simulink model "pidController"  (R2024a)
settings: Solver=VariableStepAuto  StartTime=0.0  StopTime=0.1  MaxStep=0.001  RelTol=1e-3
values from neighbouring files (symbols this model uses):
  C2 = 1e-7    (= 1e-07)    [plotPidController.m]
  C3 = 1e-6    (= 1e-06)    [plotPidController.m]
  R6 = 2e3    (= 2000)    [plotPidController.m]
settings Model: Creator=janho  LastModifiedBy=janho

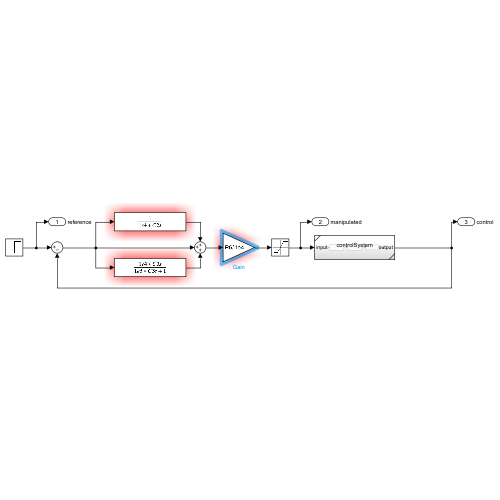
[thumbnail: Simulink's stored preview of the top-level diagram]
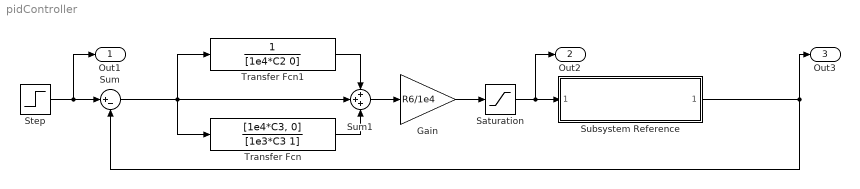
== system pidController ==
  Gain : Gain  Gain=R6/1e4
  Saturation : Saturate  UpperLimit=12  LowerLimit=-12
  Step : Step  Time=0  After=5  SampleTime=0
  Subsystem Reference : Subsystem  ReferencedSubsystem=controlSystem
  Sum : Sum  Inputs=|+-
  Sum1 : Sum  Inputs=+++
  Transfer Fcn : TransferFcn  Numerator=[1e4*C3, 0]  Denominator=[1e3*C3 1]
  Transfer Fcn1 : TransferFcn  Denominator=[1e4*C2 0]
  Out1 : Outport  SignalName=reference
  Out2 : Outport  Port=2  SignalName=manipulated
  Out3 : Outport  Port=3  SignalName=control
  wires:
  Subsystem Reference/1 -> Out3/1, Sum/2
  Step/1 -> Out1/1, Sum/1
  Saturation/1 -> Out2/1, Subsystem Reference/1
  Sum/1 -> Transfer Fcn1/1, Sum1/2, Transfer Fcn/1
  Transfer Fcn/1 -> Sum1/3
  Transfer Fcn1/1 -> Sum1/1
  Sum1/1 -> Gain/1
  Gain/1 -> Saturation/1
